simulink library "VIS_LIB_backup20190220"  (Simulink 8.6)
settings: Solver=ode45  StartTime=0.0  StopTime=10.0  RelTol=1e-3
undefined symbols (not defined in the file): AC, SIXOSEM_F_WD_AC_MASTER, VIS_LIB, WD2
libraries: cdsEpicsOut x104, cdsTP x55, cdsFilt x52, cdsFiltCtrl x23, cdsRms x23, cdsEpicsIn x16, STATE_BIO_MASTER x5, FOUROSEM_WD_AC_MASTER x4, cdsFunctionCall x2, TYPEB_MASTER x1, cdsEpicsBinIn x1, CRYP_TM_MASTER x1
(part 4 of 9)

== system VIS_LIB_backup20190220/OPLEV_BLRMS_DOF ==
  In1 : Inport
  100M_300M : cdsEpicsOut/Subsystem  Tag=cdsEpicsOutput  Description=|
      | Purpose:                                          
      | Output a FE signal to an EPICS channel.           
      |                                                   
      | Operation:                                        
      | Takes input value and passes it to EPICS record.  
      |                                                   
      | Usage:                                            
      | Name the part with the desired EPICS rrecord name.
      settings: AttributesFormatString=%<Tag>
  10_30 : cdsEpicsOut/Subsystem  Tag=cdsEpicsOutput  Description=|
      | Purpose:                                          
      | Output a FE signal to an EPICS channel.           
      |                                                   
      | Operation:                                        
      | Takes input value and passes it to EPICS record.  
      |                                                   
      | Usage:                                            
      | Name the part with the desired EPICS rrecord name.
      settings: AttributesFormatString=%<Tag>
  1_3 : cdsEpicsOut/Subsystem  Tag=cdsEpicsOutput  Description=|
      | Purpose:                                          
      | Output a FE signal to an EPICS channel.           
      |                                                   
      | Operation:                                        
      | Takes input value and passes it to EPICS record.  
      |                                                   
      | Usage:                                            
      | Name the part with the desired EPICS rrecord name.
      settings: AttributesFormatString=%<Tag>
  300M_1 : cdsEpicsOut/Subsystem  Tag=cdsEpicsOutput  Description=|
      | Purpose:                                          
      | Output a FE signal to an EPICS channel.           
      |                                                   
      | Operation:                                        
      | Takes input value and passes it to EPICS record.  
      |                                                   
      | Usage:                                            
      | Name the part with the desired EPICS rrecord name.
      settings: AttributesFormatString=%<Tag>
  30M : cdsEpicsOut/Subsystem  Tag=cdsEpicsOutput  Description=|
      | Purpose:                                          
      | Output a FE signal to an EPICS channel.           
      |                                                   
      | Operation:                                        
      | Takes input value and passes it to EPICS record.  
      |                                                   
      | Usage:                                            
      | Name the part with the desired EPICS rrecord name.
      settings: AttributesFormatString=%<Tag>
  30M_100M : cdsEpicsOut/Subsystem  Tag=cdsEpicsOutput  Description=|
      | Purpose:                                          
      | Output a FE signal to an EPICS channel.           
      |                                                   
      | Operation:                                        
      | Takes input value and passes it to EPICS record.  
      |                                                   
      | Usage:                                            
      | Name the part with the desired EPICS rrecord name.
      settings: AttributesFormatString=%<Tag>
  30_100 : cdsEpicsOut/Subsystem  Tag=cdsEpicsOutput  Description=|
      | Purpose:                                          
      | Output a FE signal to an EPICS channel.           
      |                                                   
      | Operation:                                        
      | Takes input value and passes it to EPICS record.  
      |                                                   
      | Usage:                                            
      | Name the part with the desired EPICS rrecord name.
      settings: AttributesFormatString=%<Tag>
  3_10 : cdsEpicsOut/Subsystem  Tag=cdsEpicsOutput  Description=|
      | Purpose:                                          
      | Output a FE signal to an EPICS channel.           
      |                                                   
      | Operation:                                        
      | Takes input value and passes it to EPICS record.  
      |                                                   
      | Usage:                                            
      | Name the part with the desired EPICS rrecord name.
      settings: AttributesFormatString=%<Tag>
  BLRMS : cdsFunctionCall/Subsystem  Tag=cdsFunctionCall  Description=inline BLRMS /opt/rtcds/userapps/release/cds/common/src/BLRMSFILTER.c
      settings: AttributesFormatString=%<Tag>\n%<Description>
  Constant2 : Constant  Value=2
  Demux : Demux  Outputs=8
  Mux : Mux  Inputs=2
  Terminator{1..8} (8 alike) : Terminator
  wires:
  BLRMS/1 -> Demux/1
  Mux/1 -> BLRMS/1
  In1/1 -> Mux/1
  Demux/1 -> 30M/1
  Demux/2 -> 30M_100M/1
  Demux/3 -> 100M_300M/1
  Demux/4 -> 300M_1/1
  Demux/5 -> 1_3/1
  Demux/6 -> 3_10/1
  Demux/7 -> 10_30/1
  Demux/8 -> 30_100/1
  30M/1 -> Terminator8/1
  30M_100M/1 -> Terminator1/1
  100M_300M/1 -> Terminator2/1
  300M_1/1 -> Terminator3/1
  1_3/1 -> Terminator4/1
  3_10/1 -> Terminator5/1
  10_30/1 -> Terminator6/1
  30_100/1 -> Terminator7/1
  Constant2/1 -> Mux/2

== system VIS_LIB_backup20190220/WD ==
  OSEM_UL_In : Inport
  OSEM_LL_In : Inport  Port=2
  OSEM_UR_In : Inport  Port=3
  OSEM_LR_In : Inport  Port=4
  ACT_UL_In : Inport  Port=5
  ACT_LL_In : Inport  Port=6
  ACT_UR_In : Inport  Port=7
  ACT_LR_In : Inport  Port=8
  ACT : FOUROSEM_WD_AC_MASTER/OSEMAC
  Ground5 : Ground
  OSEMAC : FOUROSEM_WD_AC_MASTER/OSEMAC
  OSEMDC : FOUROSEM_WD_DC_MASTER/OSEMDC
  RSET : cdsEpicsMomentary/EpicsMomentary  Tag=cdsEpicsMomentary
      settings: AttributesFormatString=%<Tag>
  RESET_Out : Outport
  OSEM_DC_FLAG_Out : Outport  Port=2
  OSEM_AC_FLAG_Out : Outport  Port=3
  ACT_FLAG_Out : Outport  Port=4
  wires:
  ACT/1 -> ACT_FLAG_Out/1
  ACT_LR_In/1 -> ACT/4
  ACT_UR_In/1 -> ACT/3
  OSEMAC/1 -> OSEM_AC_FLAG_Out/1
  RSET/1 -> RESET_Out/1
  OSEMDC/1 -> OSEM_DC_FLAG_Out/1
  Ground5/1 -> RSET/1
  ACT_LL_In/1 -> ACT/2
  ACT_UL_In/1 -> ACT/1
  OSEM_UL_In/1 -> OSEMDC/1, OSEMAC/1
  OSEM_LL_In/1 -> OSEMDC/2, OSEMAC/2
  OSEM_UR_In/1 -> OSEMDC/3, OSEMAC/3
  OSEM_LR_In/1 -> OSEMDC/4, OSEMAC/4

== system VIS_LIB_backup20190220/WD1 ==
  OSEM_H1_In : Inport
  OSEM_H2_In : Inport  Port=2
  OSEM_H3_In : Inport  Port=3
  OSEM_H4_In : Inport  Port=4
  OSEMAC : FOUROSEM_WD_AC_MASTER/OSEMAC
  OSEM_AC_FLAG_Out : Outport
  wires:
  OSEMAC/1 -> OSEM_AC_FLAG_Out/1
  OSEM_H1_In/1 -> OSEMAC/1
  OSEM_H3_In/1 -> OSEMAC/3
  OSEM_H2_In/1 -> OSEMAC/2
  OSEM_H4_In/1 -> OSEMAC/4

== system VIS_LIB_backup20190220/WD2 ==
  LVDT_F0_In : Inport
  LVDT_SF_In : Inport  Port=2
  LVDT_BF_In : Inport  Port=3
  AC : Subsystem
  LVDT_AC_FLAG_Out : Outport
  wires:
  AC/1(FLAG) -> LVDT_AC_FLAG_Out/1
  LVDT_BF_In/1 -> AC/3(BF_In)
  LVDT_SF_In/1 -> AC/2(SF_In)
  LVDT_F0_In/1 -> AC/1(F0_In)

== system VIS_LIB_backup20190220/WD3 ==
  OSEM_V1_In : Inport
  OSEM_V2_In : Inport  Port=2
  OSEM_V3_In : Inport  Port=3
  OSEM_H1_In : Inport  Port=4
  OSEM_H2_In : Inport  Port=5
  OSEM_H3_In : Inport  Port=6
  OSEMAC : Subsystem  AncestorBlock=SIXOSEM_F_WD_AC_MASTER/AC
  OSEM_AC_FLAG_Out : Outport
  wires:
  OSEMAC/1(FLAG) -> OSEM_AC_FLAG_Out/1
  OSEM_V1_In/1 -> OSEMAC/1(V1_In)
  OSEM_V2_In/1 -> OSEMAC/2(V2_In)
  OSEM_V3_In/1 -> OSEMAC/3(V3_In)
  OSEM_H1_In/1 -> OSEMAC/4(H1_In)
  OSEM_H2_In/1 -> OSEMAC/5(H2_In1)
  OSEM_H3_In/1 -> OSEMAC/6(H3_In1)

== system VIS_LIB_backup20190220/WD4 ==
  LVDT_SF_In : Inport
  LVDT_BF_In : Inport  Port=2
  AC : Subsystem
  LVDT_AC_FLAG_Out : Outport
  wires:
  AC/1(FLAG) -> LVDT_AC_FLAG_Out/1
  LVDT_BF_In/1 -> AC/2(BF_In)
  LVDT_SF_In/1 -> AC/1(SF_In)

== system VIS_LIB_backup20190220/WDMON ==
  BLOCK_Flag : Inport
  STATE_Flag : Inport  Port=2
  FIRST_Flag : Inport  Port=3
  CURRENT_Flag : Inport  Port=4
  BLOCK : cdsEpicsOut/Subsystem  Tag=cdsEpicsOutput  Description="field(PREC,\"3\")"
      settings: AttributesFormatString=%<Tag>
  CURRENTTRIG : cdsEpicsOut/Subsystem  Tag=cdsEpicsOutput  Description="field(PREC,\"3\")"
      settings: AttributesFormatString=%<Tag>
  FIRSTTRIG : cdsEpicsOut/Subsystem  Tag=cdsEpicsOutput  Description="field(PREC,\"3\")"
      settings: AttributesFormatString=%<Tag>
  STATE : cdsEpicsOut/Subsystem  Tag=cdsEpicsOutput  Description="field(PREC,\"3\")"
      settings: AttributesFormatString=%<Tag>
  Terminator{1,3,10..11} (4 alike) : Terminator
  wires:
  STATE_Flag/1 -> STATE/1
  FIRST_Flag/1 -> FIRSTTRIG/1
  CURRENT_Flag/1 -> CURRENTTRIG/1
  CURRENTTRIG/1 -> Terminator11/1
  FIRSTTRIG/1 -> Terminator10/1
  BLOCK_Flag/1 -> BLOCK/1
  BLOCK/1 -> Terminator1/1
  STATE/1 -> Terminator3/1

== system VIS_LIB_backup20190220/WD_BF ==
  LVDT_GAS_In : Inport
  LVDT_V1_In : Inport  Port=2
  LVDT_V2_In : Inport  Port=3
  LVDT_V3_In : Inport  Port=4
  LVDT_H1_In : Inport  Port=5
  LVDT_H2_In : Inport  Port=6
  LVDT_H3_In : Inport  Port=7
  AC : BF_WD_MASTER/AC
  AC_FLAG_Out : Outport
  wires:
  AC/1 -> AC_FLAG_Out/1
  LVDT_GAS_In/1 -> AC/1
  LVDT_V1_In/1 -> AC/2
  LVDT_V2_In/1 -> AC/3
  LVDT_V3_In/1 -> AC/4
  LVDT_H1_In/1 -> AC/5
  LVDT_H2_In/1 -> AC/6
  LVDT_H3_In/1 -> AC/7

== system VIS_LIB_backup20190220/WD_GAS ==
  GAS_In : Inport
  AC : GAS_WD_MASTER/GASAC
  GAS_AC_FLAG_Out : Outport
  wires:
  AC/1 -> GAS_AC_FLAG_Out/1
  GAS_In/1 -> AC/1

== system VIS_LIB_backup20190220/WD_TEST4CH ==
  SEN1_In : Inport
  SEN2_In : Inport  Port=2
  SEN3_In : Inport  Port=3
  SEN4_In : Inport  Port=4
  OSEMAC : FOUROSEM_WD_AC_MASTER/OSEMAC
  TESTSEN_AC_FLAG_Out : Outport
  wires:
  OSEMAC/1 -> TESTSEN_AC_FLAG_Out/1
  SEN1_In/1 -> OSEMAC/1
  SEN3_In/1 -> OSEMAC/3
  SEN2_In/1 -> OSEMAC/2
  SEN4_In/1 -> OSEMAC/4

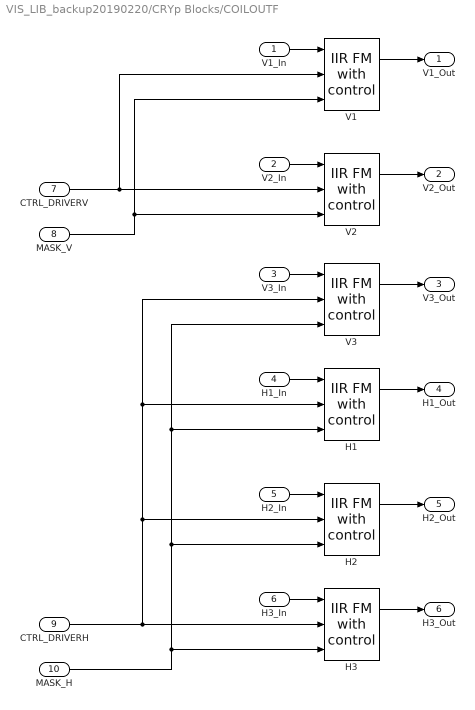
== system VIS_LIB_backup20190220/CRYp Blocks/COILOUTF ==
  V1_In : Inport
  V2_In : Inport  Port=2
  V3_In : Inport  Port=3
  H1_In : Inport  Port=4
  H2_In : Inport  Port=5
  H3_In : Inport  Port=6
  CTRL_DRIVERV : Inport  Port=7
  MASK_V : Inport  Port=8
  CTRL_DRIVERH : Inport  Port=9
  MASK_H : Inport  Port=10
  H1 : cdsFiltCtrl/IIR FM with control  Tag=cdsFiltCtrl  Description=|
      | cdsFiltCntrl is the standard IIR filter module (exactly the same as cdsFilt) but with added control data output 'Ctrl'. Filter module digital signal output appears on the first output, which is called 'Val'. 'Ctrl' output has a bit pattern encoding the state of filter's on/off switches (FM1 through FM10). The bit values are:
      |                                                                                                                                                                                                                                                                                                                                       
      | module 	hex	dec                                                                                                                                                                                                                                                                                                                       
      | -----------------------                                                                                                                                                                                                                                                                                                               
      | FM1	0x20                    32                                                                                                                                                                                                                                                                                                        
      | FM2	0x80                     128                                                                                                                                                                                                                                                                                                      
      | FM3	0x200                   512                                                                                                                                                                                                                                                                                                       
      | FM4	0x800                   2048                                                                                                                                                                                                                                                                                                      
      | FM5	0x2000                 8192                                                                                                                                                                                                                                                                                                       
      | FM6	0x8000                 32768                                                                                                                                                                                                                                                                                                      
      | FM7	0x20000                131072                                                                                                                                                                                                                                                                                                     
      | FM8	0x80000                 524288                                                                                                                                                                                                                                                                                                    
      | FM9	0x200000               2097152                                                                                                                                                                                                                                                                                                    
      | FM10	0x800000               8388608                                                                                                                                                                                                                                                                                                   
      |                                                                                                                                                                                                                                                                                                                                       
      | This bit data can be used to drive some other switches or it can be output using a binary I/O module.
      settings: AttributesFormatString=%<Tag>
  H2 : cdsFiltCtrl/IIR FM with control  Tag=cdsFiltCtrl  Description=|
      | cdsFiltCntrl is the standard IIR filter module (exactly the same as cdsFilt) but with added control data output 'Ctrl'. Filter module digital signal output appears on the first output, which is called 'Val'. 'Ctrl' output has a bit pattern encoding the state of filter's on/off switches (FM1 through FM10). The bit values are:
      |                                                                                                                                                                                                                                                                                                                                       
      | module 	hex	dec                                                                                                                                                                                                                                                                                                                       
      | -----------------------                                                                                                                                                                                                                                                                                                               
      | FM1	0x20                    32                                                                                                                                                                                                                                                                                                        
      | FM2	0x80                     128                                                                                                                                                                                                                                                                                                      
      | FM3	0x200                   512                                                                                                                                                                                                                                                                                                       
      | FM4	0x800                   2048                                                                                                                                                                                                                                                                                                      
      | FM5	0x2000                 8192                                                                                                                                                                                                                                                                                                       
      | FM6	0x8000                 32768                                                                                                                                                                                                                                                                                                      
      | FM7	0x20000                131072                                                                                                                                                                                                                                                                                                     
      | FM8	0x80000                 524288                                                                                                                                                                                                                                                                                                    
      | FM9	0x200000               2097152                                                                                                                                                                                                                                                                                                    
      | FM10	0x800000               8388608                                                                                                                                                                                                                                                                                                   
      |                                                                                                                                                                                                                                                                                                                                       
      | This bit data can be used to drive some other switches or it can be output using a binary I/O module.
      settings: AttributesFormatString=%<Tag>
  H3 : cdsFiltCtrl/IIR FM with control  Tag=cdsFiltCtrl  Description=|
      | cdsFiltCntrl is the standard IIR filter module (exactly the same as cdsFilt) but with added control data output 'Ctrl'. Filter module digital signal output appears on the first output, which is called 'Val'. 'Ctrl' output has a bit pattern encoding the state of filter's on/off switches (FM1 through FM10). The bit values are:
      |                                                                                                                                                                                                                                                                                                                                       
      | module 	hex	dec                                                                                                                                                                                                                                                                                                                       
      | -----------------------                                                                                                                                                                                                                                                                                                               
      | FM1	0x20                    32                                                                                                                                                                                                                                                                                                        
      | FM2	0x80                     128                                                                                                                                                                                                                                                                                                      
      | FM3	0x200                   512                                                                                                                                                                                                                                                                                                       
      | FM4	0x800                   2048                                                                                                                                                                                                                                                                                                      
      | FM5	0x2000                 8192                                                                                                                                                                                                                                                                                                       
      | FM6	0x8000                 32768                                                                                                                                                                                                                                                                                                      
      | FM7	0x20000                131072                                                                                                                                                                                                                                                                                                     
      | FM8	0x80000                 524288                                                                                                                                                                                                                                                                                                    
      | FM9	0x200000               2097152                                                                                                                                                                                                                                                                                                    
      | FM10	0x800000               8388608                                                                                                                                                                                                                                                                                                   
      |                                                                                                                                                                                                                                                                                                                                       
      | This bit data can be used to drive some other switches or it can be output using a binary I/O module.
      settings: AttributesFormatString=%<Tag>
  V1 : cdsFiltCtrl/IIR FM with control  Tag=cdsFiltCtrl  Description=|
      | cdsFiltCntrl is the standard IIR filter module (exactly the same as cdsFilt) but with added control data output 'Ctrl'. Filter module digital signal output appears on the first output, which is called 'Val'. 'Ctrl' output has a bit pattern encoding the state of filter's on/off switches (FM1 through FM10). The bit values are:
      |                                                                                                                                                                                                                                                                                                                                       
      | module 	hex	dec                                                                                                                                                                                                                                                                                                                       
      | -----------------------                                                                                                                                                                                                                                                                                                               
      | FM1	0x20                    32                                                                                                                                                                                                                                                                                                        
      | FM2	0x80                     128                                                                                                                                                                                                                                                                                                      
      | FM3	0x200                   512                                                                                                                                                                                                                                                                                                       
      | FM4	0x800                   2048                                                                                                                                                                                                                                                                                                      
      | FM5	0x2000                 8192                                                                                                                                                                                                                                                                                                       
      | FM6	0x8000                 32768                                                                                                                                                                                                                                                                                                      
      | FM7	0x20000                131072                                                                                                                                                                                                                                                                                                     
      | FM8	0x80000                 524288                                                                                                                                                                                                                                                                                                    
      | FM9	0x200000               2097152                                                                                                                                                                                                                                                                                                    
      | FM10	0x800000               8388608                                                                                                                                                                                                                                                                                                   
      |                                                                                                                                                                                                                                                                                                                                       
      | This bit data can be used to drive some other switches or it can be output using a binary I/O module.
      settings: AttributesFormatString=%<Tag>
  V2 : cdsFiltCtrl/IIR FM with control  Tag=cdsFiltCtrl  Description=|
      | cdsFiltCntrl is the standard IIR filter module (exactly the same as cdsFilt) but with added control data output 'Ctrl'. Filter module digital signal output appears on the first output, which is called 'Val'. 'Ctrl' output has a bit pattern encoding the state of filter's on/off switches (FM1 through FM10). The bit values are:
      |                                                                                                                                                                                                                                                                                                                                       
      | module 	hex	dec                                                                                                                                                                                                                                                                                                                       
      | -----------------------                                                                                                                                                                                                                                                                                                               
      | FM1	0x20                    32                                                                                                                                                                                                                                                                                                        
      | FM2	0x80                     128                                                                                                                                                                                                                                                                                                      
      | FM3	0x200                   512                                                                                                                                                                                                                                                                                                       
      | FM4	0x800                   2048                                                                                                                                                                                                                                                                                                      
      | FM5	0x2000                 8192                                                                                                                                                                                                                                                                                                       
      | FM6	0x8000                 32768                                                                                                                                                                                                                                                                                                      
      | FM7	0x20000                131072                                                                                                                                                                                                                                                                                                     
      | FM8	0x80000                 524288                                                                                                                                                                                                                                                                                                    
      | FM9	0x200000               2097152                                                                                                                                                                                                                                                                                                    
      | FM10	0x800000               8388608                                                                                                                                                                                                                                                                                                   
      |                                                                                                                                                                                                                                                                                                                                       
      | This bit data can be used to drive some other switches or it can be output using a binary I/O module.
      settings: AttributesFormatString=%<Tag>
  V3 : cdsFiltCtrl/IIR FM with control  Tag=cdsFiltCtrl  Description=|
      | cdsFiltCntrl is the standard IIR filter module (exactly the same as cdsFilt) but with added control data output 'Ctrl'. Filter module digital signal output appears on the first output, which is called 'Val'. 'Ctrl' output has a bit pattern encoding the state of filter's on/off switches (FM1 through FM10). The bit values are:
      |                                                                                                                                                                                                                                                                                                                                       
      | module 	hex	dec                                                                                                                                                                                                                                                                                                                       
      | -----------------------                                                                                                                                                                                                                                                                                                               
      | FM1	0x20                    32                                                                                                                                                                                                                                                                                                        
      | FM2	0x80                     128                                                                                                                                                                                                                                                                                                      
      | FM3	0x200                   512                                                                                                                                                                                                                                                                                                       
      | FM4	0x800                   2048                                                                                                                                                                                                                                                                                                      
      | FM5	0x2000                 8192                                                                                                                                                                                                                                                                                                       
      | FM6	0x8000                 32768                                                                                                                                                                                                                                                                                                      
      | FM7	0x20000                131072                                                                                                                                                                                                                                                                                                     
      | FM8	0x80000                 524288                                                                                                                                                                                                                                                                                                    
      | FM9	0x200000               2097152                                                                                                                                                                                                                                                                                                    
      | FM10	0x800000               8388608                                                                                                                                                                                                                                                                                                   
      |                                                                                                                                                                                                                                                                                                                                       
      | This bit data can be used to drive some other switches or it can be output using a binary I/O module.
      settings: AttributesFormatString=%<Tag>
  V1_Out : Outport
  V2_Out : Outport  Port=2
  V3_Out : Outport  Port=3
  H1_Out : Outport  Port=4
  H2_Out : Outport  Port=5
  H3_Out : Outport  Port=6
  wires:
  MASK_H/1 -> H1/3, V3/3, H2/3, H3/3
  CTRL_DRIVERH/1 -> H1/2, V3/2, H2/2, H3/2
  MASK_V/1 -> V1/3, V2/3
  CTRL_DRIVERV/1 -> V1/2, V2/2
  V1/1 -> V1_Out/1
  V1_In/1 -> V1/1
  V2_In/1 -> V2/1
  V2/1 -> V2_Out/1
  V3_In/1 -> V3/1
  V3/1 -> V3_Out/1
  H1_In/1 -> H1/1
  H1/1 -> H1_Out/1
  H2_In/1 -> H2/1
  H2/1 -> H2_Out/1
  H3_In/1 -> H3/1
  H3/1 -> H3_Out/1
